simulink model "StepResponce"  (R2020b)
settings: Solver=VariableStepAuto  StartTime=0.0  StopTime=600  RelTol=1e-3
libraries: realtime_pacer_lib x1
settings Model: Creator=diego  LastModifiedBy=diego

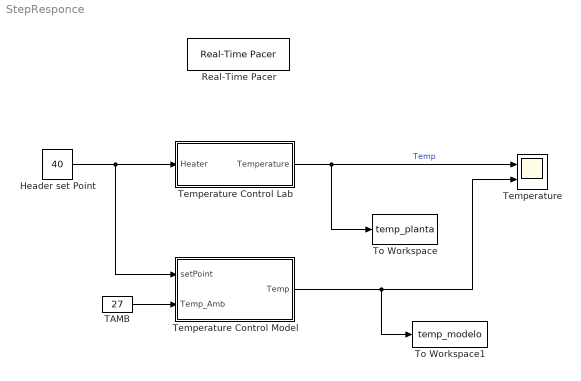
== system StepResponce ==
  Header set Point : Constant  Value=40
  Real-Time Pacer : realtime_pacer_lib/Real-Time Pacer  simTimePerRealTime=1
  TAMB : Constant  Value=27
  Temperature : Scope  NumInputPorts=2
  Temperature Control Lab : Subsystem
  Temperature Control Model : Subsystem
  To Workspace : ToWorkspace  VariableName=temp_planta  SampleTime=1
      settings: Save2DSignal=2-D array (concatenate along first dimension)
  To Workspace1 : ToWorkspace  VariableName=temp_modelo  SampleTime=1
      settings: Save2DSignal=2-D array (concatenate along first dimension)
  wires:
  Temperature Control Lab/1(Temperature) -> To Workspace/1, Temperature/1  "Temp"
  Header set Point/1 -> Temperature Control Model/1(setPoint), Temperature Control Lab/1(Heater)
  Temperature Control Model/1(Temp) -> To Workspace1/1, Temperature/2
  TAMB/1 -> Temperature Control Model/2(Temp_Amb)

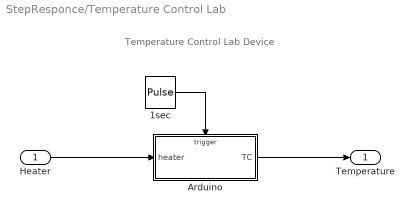
== system StepResponce/Temperature Control Lab ==
  note: Temperature Control Lab Device
  Heater : Inport
  1sec : DiscretePulseGenerator  PulseType=Time based  Period=1  PulseWidth=50
  Arduino : Subsystem  TreatAsAtomicUnit=on
  Temperature : Outport  VectorParamsAs1DForOutWhenUnconnected=off
  wires:
  1sec/1 -> Arduino/Trigger
  Arduino/1(TC) -> Temperature/1
  Heater/1 -> Arduino/1(heater)

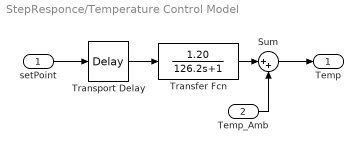
== system StepResponce/Temperature Control Model ==
  setPoint : Inport
  Temp_Amb : Inport  Port=2
  Sum : Sum  Inputs=|++
  Transfer Fcn : TransferFcn  Numerator=[1.20]  Denominator=[126.2, 1]
  Transport Delay : TransportDelay  DelayTime=14.23
  Temp : Outport
  wires:
  Transport Delay/1 -> Transfer Fcn/1
  Temp_Amb/1 -> Sum/2
  Sum/1 -> Temp/1
  Transfer Fcn/1 -> Sum/1
  setPoint/1 -> Transport Delay/1

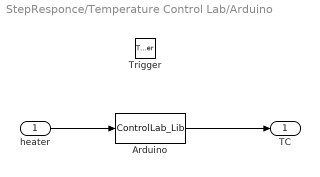
== system StepResponce/Temperature Control Lab/Arduino ==
  heater : Inport  LatchByDelayingOutsideSignal=on
  Trigger : TriggerPort  VariantControl=Variant
  Arduino : MATLABFcn  MATLABFcn=ControlLab_Lib
  TC : Outport  InitialOutput=23  VectorParamsAs1DForOutWhenUnconnected=off
  wires:
  heater/1 -> Arduino/1
  Arduino/1 -> TC/1
